simulink model "control_sim_hw3"  (R2023b)
settings: Solver=ode4  StartTime=0.0  StopTime=20  RelTol=1e-3
settings Model: Creator=henry  LastModifiedBy=henry

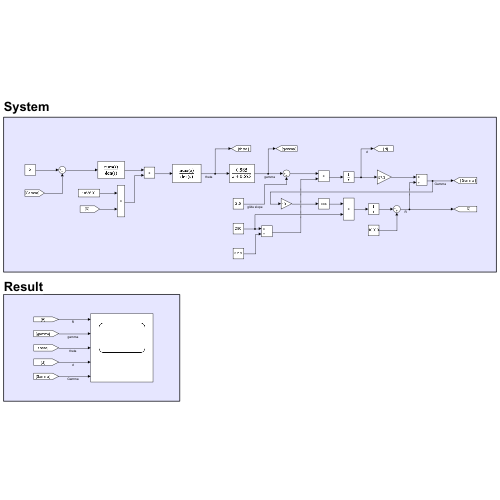
[thumbnail: Simulink's stored preview of the top-level diagram]
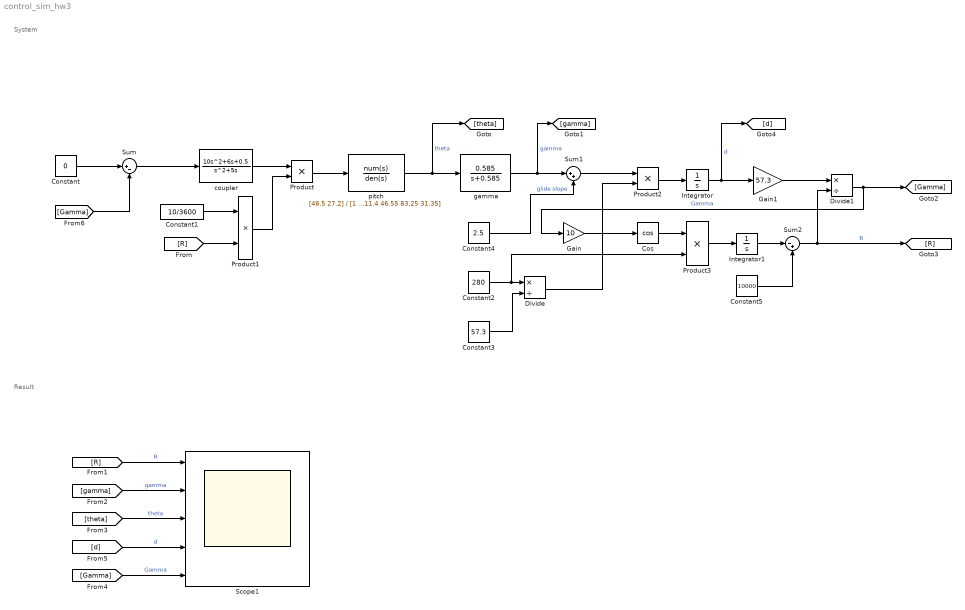
== system control_sim_hw3 ==
  note: Result
  note: System
  Constant : Constant  Value=0
  Constant1 : Constant  Value=10/3600
  Constant2 : Constant  Value=280
  Constant3 : Constant  Value=57.3
  Constant4 : Constant  Value=2.5
  Constant5 : Constant  Value=10000
  Cos : Trigonometry  Operator=cos
  Divide : Product  Inputs=*/
  Divide1 : Product  Inputs=*/
  Gain : Gain  Gain=10
  Gain1 : Gain  Gain=57.3
  Integrator : Integrator
  Integrator1 : Integrator
  Product{,1..3} (4 alike) : Product
  Scope1 : Scope  NumInputPorts=5
  Sum : Sum  Inputs=|+-
  Sum1 : Sum  Inputs=|++
  Sum2 : Sum  Inputs=|-+
  coupler : TransferFcn  Numerator=[10 6 0.5]  Denominator=[1 5 0]
  gamma : TransferFcn  Numerator=[0.585]  Denominator=[1 0.585]
  pitch : TransferFcn  Numerator=[46.5 27.2]  Denominator=[1 11.4 46.55 83.25 31.35]
  wires:
  [R] -> Scope1/1  "R"
  [gamma] -> Scope1/2  "gamma"
  [theta] -> Scope1/3  "theta"
  [d] -> Scope1/4  "d"
  [Gamma] -> Scope1/5  "Gamma"
  Product/1 -> pitch/1
  pitch/1 -> gamma/1, [theta]  "theta"
  Gain/1 -> Cos/1
  Constant5/1 -> Sum2/2
  Constant1/1 -> Product1/1
  Product2/1 -> Integrator/1
  Sum/1 -> coupler/1
  Constant3/1 -> Divide/2
  Divide/1 -> Product2/2
  Divide1/1 -> Gain/1, [Gamma]  "Gamma"
  gamma/1 -> Sum1/1, [gamma]  "gamma"
  coupler/1 -> Product/1
  Integrator/1 -> Gain1/1, [d]  "d"
  Constant2/1 -> Product3/2, Divide/1
  Sum1/1 -> Product2/1
  Product1/1 -> Product/2
  Cos/1 -> Product3/1
  [Gamma] -> Sum/2
  Constant/1 -> Sum/1
  Constant4/1 -> Sum1/2  "glide slope"
  Gain1/1 -> Divide1/1
  Sum2/1 -> [R], Divide1/2  "R"
  Integrator1/1 -> Sum2/1
  Product3/1 -> Integrator1/1
  [R] -> Product1/2
